simulink model "Models_for_report"  (R2015b)
settings: Solver=VariableStepAuto  StartTime=0.0  StopTime=10.0  RelTol=1e-3
values from neighbouring files (symbols this model uses):
  J_pro = (m*r^2+J_G2)*(G1/G2)^2 + J_G1    (= 0.281547798877)    [Control_Parameters.m]    (also in M_fil_til_jacob.m; PMSM_State_Space_Parameters.m)
  Kt = .07329    (= 0.07329)    [Control_Parameters.m]    (also in M_fil_til_jacob.m; PMSM_State_Space_Parameters.m)
  Kv = 0.001    [Control_Parameters.m]    (also in M_fil_til_jacob.m)
  R = .013/2    (= 0.0065)    [Control_Parameters.m]    (also in M_fil_til_jacob.m; PMSM_State_Space_Parameters.m)
  TS = L/R    (= 0.00615384615385)    [Control_Parameters.m]    (also in M_fil_til_jacob.m; PMSM_State_Space_Parameters.m)
undefined symbols (not defined in the file or in its folder): C_drag, T_L
settings Model: Creator=Morten  LastModifiedBy=Morten

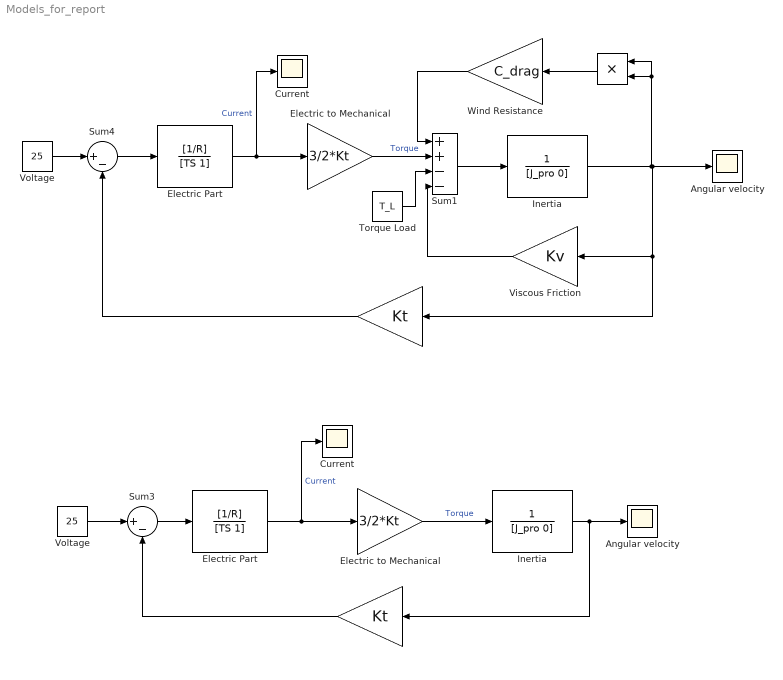
== system Models_for_report ==
  "           " : Product
  "            " : Gain  Gain=Kt
  "             " : Gain  Gain=Kt
  Angular velocity : Scope
  "Angular velocity " : Scope
  Current : Scope
  "Current " : Scope
  Electric Part : TransferFcn  Numerator=[1/R]  Denominator=[TS 1]
  "Electric Part " : TransferFcn  Numerator=[1/R]  Denominator=[TS 1]
  Electric to Mechanical : Gain  Gain=3/2*Kt
  "Electric to Mechanical " : Gain  Gain=3/2*Kt
  Inertia : TransferFcn  Denominator=[J_pro 0]
  "Inertia " : TransferFcn  Denominator=[J_pro 0]
  Sum1 : Sum  Inputs=++--
  Sum3 : Sum  Inputs=|+-
  Sum4 : Sum  Inputs=|+-
  Torque Load : Constant  Value=T_L
  Viscous Friction : Gain  Gain=Kv
  Voltage : Constant  Value=25
  "Voltage " : Constant  Value=25
  Wind Resistance : Gain  Gain=C_drag
  wires:
  "            "/1 -> Sum4/2
  Sum4/1 -> Electric Part/1
  Electric Part/1 -> Current/1, Electric to Mechanical/1  "Current"
  "           "/1 -> Wind Resistance/1
  Voltage/1 -> Sum4/1
  Electric to Mechanical/1 -> Sum1/2  "Torque"
  Sum1/1 -> Inertia/1
  Wind Resistance/1 -> Sum1/1
  Torque Load/1 -> Sum1/3
  Viscous Friction/1 -> Sum1/4
  Inertia/1 -> Angular velocity/1, Viscous Friction/1, "            "/1, "           "/1, "           "/2
  "             "/1 -> Sum3/2
  Sum3/1 -> "Electric Part "/1
  "Electric Part "/1 -> "Current "/1, "Electric to Mechanical "/1  "Current"
  "Voltage "/1 -> Sum3/1
  "Electric to Mechanical "/1 -> "Inertia "/1  "Torque"
  "Inertia "/1 -> "Angular velocity "/1, "             "/1
